simulink model "sim2_CompleteModel"  (R2014a)
settings: Solver=ode4  StartTime=0  StopTime=25  FixedStep=0.001  RelTol=1e-3
libraries: simulink x1
settings Model: Creator=Bruno  LastModifiedBy=Bruno
settings SolverCC: MaxConsecutiveZCs=100  ZeroCrossAlgorithm=Adaptive

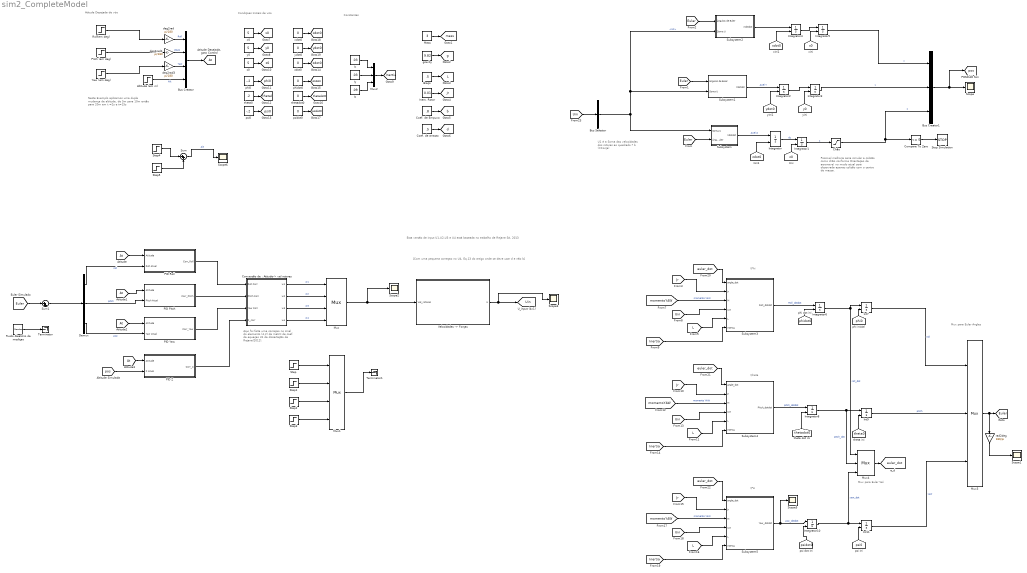
== system sim2_CompleteModel ==
  note: Aqui foi feita uma correçao no sinal do elemento (4,2) da matriz de coef. da equaçao 31 da dissertação de Rejane(2012).
  note: Neste Exemplo aplicamos uma dupla mudança de altitude, de 5m para 10m então para 20m em t =2s e t=15s
  note: Atitude Desejada de vôo
  note: Possível melhoria seria simular a colisão como chão conforme Orientaçao da aeronave! no modo atual será observada apenas colisão com o centro de massa.
  note: U1 é a Soma das velocidades dos rotores ao quadrado * b (=Força)
  note: \theta
  note: Mux para Euler Angles
  note: [Com uma pequena correçao no U4, Eq.13 do artigo onde se deve usar d e não b]
  note: Esta versão de input U1,U2,U3 e U4 está baseada no trabalho de Rejane Sá, 2013
  note: Constantes
  note: \Phi
  note: \Psi
  note: Mux para Euler Vel.
  note: Condiçoes Iniciais de vôo
  Altitude (em m) : Step  Time=0  Before=5  After=5  SampleTime=0
  Braço : Constant  Value=.5
  Bus Creator : BusCreator
  Bus Creator1 : BusCreator  Inputs=3
  Bus Selector : BusSelector  OutputSignals=U1
  Chão : Saturate  UpperLimit=inf  LowerLimit=-0.01
  Coef. de Empuxo : Constant  Value=.8
  Coef. de arrasto : Constant  Value=.5
  Compare To Zero : simulink/Logic and Bit Operations/Compare To Zero  relop=<=  OutDataTypeStr=boolean
  "Conversão de : Atitude-> vel rotores" : Subsystem
  Demux : Demux  Outputs=3
  Inerc. Rotor : Constant  Value=0.01
  Int11 : Integrator  InitialConditionSource=external
  Int7 : Integrator  InitialConditionSource=external
  Int9 : Integrator  InitialConditionSource=external
  Integrator : Integrator  InitialConditionSource=external  UpperSaturationLimit=1  LowerSaturationLimit=-1  IgnoreLimit=on
  Integrator1 : Integrator  InitialConditionSource=external  InitialCondition=20
  Integrator10 : Integrator  InitialConditionSource=external  UpperSaturationLimit=1  LowerSaturationLimit=-1  IgnoreLimit=on
  Integrator{2..6,8} (6 alike) : Integrator  InitialConditionSource=external
  Ix : Constant  Value=.03
  Iy : Constant  Value=.03
  Iz : Constant  Value=.09
  Mass : Constant  Value=3
  Mux : Mux
      settings: DisplayOption=signals
  Mux1 : Mux
      settings: DisplayOption=signals
  Mux2 : Mux  Inputs=3
  Mux3 : Mux  Inputs=3
      settings: DisplayOption=signals
  Mux4 : Mux  Inputs=3
      settings: DisplayOption=signals
  PID Pitch : Subsystem
  PID Roll : Subsystem
  PID Yaw : Subsystem
  PID Z : Subsystem
  Pitch (em deg) : Step  Time=0  After=0  SampleTime=0
  Roll(em deg) : Step  Time=0  After=0  SampleTime=0
  Ruído Aleatório da mediçao : UniformRandomNumber  Minimum=-.005  Maximum=.005  SampleTime=0
  Scope{,1..3,5..6} (6 alike) : Scope
      Scope settings: ShowLegends=on  YMin=3.95  SaveName=XYZ_Strategy1_C
      Scope1 settings: SaveName=Euler_Strategy1_C  Decimation=100
      Scope2 settings: ShowLegends=on  YMin=-1.1e+07  YMax=1.1e+07  SaveName=ScopeData3
      Scope3 settings: ShowLegends=on  YMin=0  YMax=1.3e+07  SaveName=ScopeData6
      Scope5 settings: ShowLegends=on  SaveName=ScopeData11
      Scope6 settings: ShowLegends=on  SaveName=ScopeData12
  Step{,1..3} (4 alike) : Step  Time=0  After=15  SampleTime=0
  Step4 : Step  Time=0  Before=5  After=5  SampleTime=0
  Step5 : Step  Time=5  SampleTime=0
  Stop Simulation : Stop
  Subsystem : Subsystem
  Subsystem1 : Subsystem
  Subsystem2 : Subsystem
  Subsystem3 : Subsystem
  Subsystem4 : Subsystem
  Subsystem5 : Subsystem
  Sum : Sum  Inputs=|++
  Sum1 : Sum  Inputs=|++
  Terminator : Terminator
  Terminator1 : Terminator
  "Velocidades -> Forças" : Subsystem
  Yaw (em deg) : Step  Time=0  After=0  SampleTime=0
  deg2rad : Gain  Gain=pi/180
  deg2rad2 : Gain  Gain=pi/180
  deg2rad3 : Gain  Gain=pi/180
  gravity : Constant  Value=9.82
  phi0 : Constant  Value=-.2
  phidot0 : Constant  Value=0
  psi0 : Constant  Value=-.2
  psidot0 : Constant  Value=0
  rad2deg : Gain  Gain=180/pi
  theta0 : Constant  Value=.2
  thetadot0 : Constant  Value=0
  x0 : Constant  Value=5
  xdot0 : Constant  Value=0
  y0 : Constant  Value=5
  ydot0 : Constant  Value=0
  z0 : Constant  Value=5
  zdot0 : Constant  Value=0
  tag scope: At=global, Euler=global, Inertia=global, Jr=global, L=global, Uin=global, b=global, d=global, euler_dot=global, g=global, mass=global, phi0=global, phidot0=global, pos=global, psi0=global, psidot0=global, theta0=global, thetadot0=global, x0=global, xdot0=global, y0=global, ydot0=global, z0=global, zdot0=global
  wires:
  Integrator/1 -> Integrator1/1  "dz"
  Integrator1/1 -> Chão/1  "z"
  Subsystem/1(zdotdot) -> Integrator/1  "Acel Z"
  Bus Selector/1 -> Subsystem/1(Soma U), Subsystem2/2(Soma U), Subsystem1/2(Soma U)  "<U1>"
  Subsystem1/1(Ydotdot) -> Integrator2/1  "Acel Y"
  Integrator2/1 -> Integrator3/1
  Subsystem2/1(Xdotdot) -> Integrator4/1
  Integrator4/1 -> Integrator5/1
  [Euler] -> Subsystem/2(Ângulos de Euler)
  [Euler] -> Subsystem1/1(ângulos de Euler)
  [Euler] -> Subsystem2/1(ângulos de Euler)
  Mass/1 -> [mass]
  gravity/1 -> [g]
  Braço/1 -> [L]
  [euler_dot] -> Subsystem3/1(angle_dot)
  [Jr] -> Subsystem3/2(Jr)
  [momentoYAW] -> Subsystem3/3(M)  "momento YAW"
  [Uin] -> Subsystem3/4(Uin)
  [L] -> Subsystem3/5(L)
  [Inertia] -> Subsystem3/6(Inertia)
  Subsystem3/1(Roll_dotdot) -> Integrator6/1  "Roll_dotdot"
  Inerc. Rotor/1 -> [Jr]
  Coef. de Empuxo/1 -> [b]
  Coef. de arrasto/1 -> [d]
  Iy/1 -> Mux2/2
  Ix/1 -> Mux2/1
  Iz/1 -> Mux2/3
  Mux2/1 -> [Inertia]
  Integrator6/1 -> Int7/1, Mux4/1  "roll_dot"
  Int7/1 -> Mux3/1  "roll"
  Mux3/1 -> [Euler], rad2deg/1
  [euler_dot] -> Subsystem4/1(angle_dot)
  [Jr] -> Subsystem4/2(Jr)
  [momentoYAW] -> Subsystem4/3(M)  "momento YAW"
  [Uin] -> Subsystem4/4(Uin)
  [L] -> Subsystem4/5(L)
  [Inertia] -> Subsystem4/6(Inertia)
  Subsystem4/1(Pitch_dotdot) -> Integrator8/1  "pitch_dotdot"
  Integrator8/1 -> Mux4/2, Int9/1  "pitch_dot"
  Int9/1 -> Mux3/2  "pitch"
  [euler_dot] -> Subsystem5/1(angle_dot)
  [Jr] -> Subsystem5/2(Jr)
  [momentoYAW] -> Subsystem5/3(M)  "momento YAW"
  [Uin] -> Subsystem5/4(Uin)
  [L] -> Subsystem5/5(L)
  [Inertia] -> Subsystem5/6(Inertia)
  Subsystem5/1(Yaw_dotdot) -> Scope5/1, Integrator10/1  "yaw_dotdot"
  Integrator10/1 -> Mux4/3, Int11/1  "yaw_dot"
  Int11/1 -> Mux3/3  "yaw"
  Mux4/1 -> [euler_dot]
  [Uin] -> Bus Selector/1
  Integrator3/1 -> Bus Creator1/2  "y"
  "Velocidades -> Forças"/1(U) -> Scope3/1, [Uin]
  [phi0] -> Int7/2
  [psi0] -> Int11/2
  [theta0] -> Int9/2
  x0/1 -> [x0]
  theta0/1 -> [theta0]
  psi0/1 -> [psi0]
  phi0/1 -> [phi0]
  z0/1 -> [z0]
  y0/1 -> [y0]
  xdot0/1 -> [xdot0]
  thetadot0/1 -> [thetadot0]
  psidot0/1 -> [psidot0]
  phidot0/1 -> [phidot0]
  zdot0/1 -> [zdot0]
  ydot0/1 -> [ydot0]
  [z0] -> Integrator1/2
  [phidot0] -> Integrator6/2
  [thetadot0] -> Integrator8/2
  [psidot0] -> Integrator10/2
  [zdot0] -> Integrator/2
  "Conversão de : Atitude-> vel rotores"/1(w1) -> Mux/1  "w1"
  "Conversão de : Atitude-> vel rotores"/3(w3) -> Mux/3  "w3"
  "Conversão de : Atitude-> vel rotores"/2(w2) -> Mux/2  "w2"
  "Conversão de : Atitude-> vel rotores"/4(w4) -> Mux/4  "w4"
  Chão/1 -> Bus Creator1/3, Compare To Zero/1  "z"
  Compare To Zero/1 -> Stop Simulation/1
  Roll(em deg)/1 -> deg2rad/1
  Pitch (em deg)/1 -> deg2rad2/1
  Yaw (em deg)/1 -> deg2rad3/1
  Bus Creator/1 -> [At]
  deg2rad/1 -> Bus Creator/1  "Roll"
  deg2rad2/1 -> Bus Creator/2  "Pitch"
  deg2rad3/1 -> Bus Creator/3  "Yaw"
  [At] -> PID Roll/1(Atitude)
  Demux/1 -> PID Roll/2(Roll Atual)  "roll"
  [At] -> PID Pitch/1(Atitude)
  Demux/2 -> PID Pitch/2(Pitch Atual)  "pitch"
  Demux/3 -> PID Yaw/2(Yaw Atual)  "yaw"
  [At] -> PID Yaw/1(Atitude)
  [At] -> PID Z/1(Atitude)
  Bus Creator1/1 -> [pos], Scope/1
  [pos] -> PID Z/2(Z Atual)
  PID Roll/1(Corr_Roll) -> "Conversão de : Atitude-> vel rotores"/1(Roll Corr)
  PID Pitch/1(Corr_Pitch) -> "Conversão de : Atitude-> vel rotores"/2(Pitch Corr)
  PID Yaw/1(Corr_Yaw) -> "Conversão de : Atitude-> vel rotores"/3(Yaw Corr)
  PID Z/1(Corr_Z) -> "Conversão de : Atitude-> vel rotores"/4(Z_corr)
  Step4/1 -> Sum/1
  Step5/1 -> Sum/2
  Sum/1 -> Scope6/1  "Alt"
  Altitude (em m)/1 -> Bus Creator/4  "Alt"
  Integrator5/1 -> Bus Creator1/1  "x"
  [x0] -> Integrator5/2
  [xdot0] -> Integrator4/2
  [ydot0] -> Integrator2/2
  [y0] -> Integrator3/2
  Mux/1 -> "Velocidades -> Forças"/1(Vel_rotores), Scope2/1
  rad2deg/1 -> Scope1/1
  [Euler] -> Sum1/1
  Ruído Aleatório da mediçao/1 -> Terminator/1
  Sum1/1 -> Demux/1
  Step2/1 -> Mux1/3
  Step1/1 -> Mux1/2
  Step/1 -> Mux1/1
  Step3/1 -> Mux1/4
  Mux1/1 -> Terminator1/1

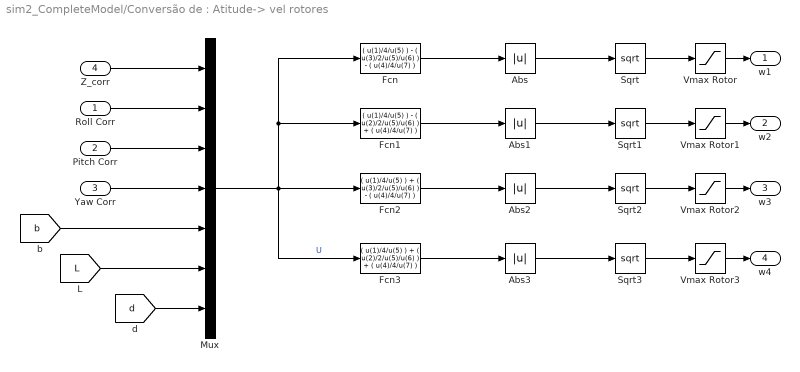
== system sim2_CompleteModel/Conversão de : Atitude-> vel rotores ==
  Roll Corr : Inport
  Pitch Corr : Inport  Port=2
  Yaw Corr : Inport  Port=3
  Z_corr : Inport  Port=4
  Abs{,1..3} (4 alike) : Abs
  Fcn : Fcn  Expr="( u(1)/4/u(5) ) - ( u(3)/2/u(5)/u(6) )  - ( u(4)/4/u(7) )"
  Fcn1 : Fcn  Expr="( u(1)/4/u(5) ) - ( u(2)/2/u(5)/u(6) )  + ( u(4)/4/u(7) )"
  Fcn2 : Fcn  Expr="( u(1)/4/u(5) ) + ( u(3)/2/u(5)/u(6) )  - ( u(4)/4/u(7) )"
  Fcn3 : Fcn  Expr="( u(1)/4/u(5) ) + ( u(2)/2/u(5)/u(6) )  + ( u(4)/4/u(7) )"
  Mux : Mux  Inputs=7
  Sqrt{,1..3} (4 alike) : Sqrt  SaturateOnIntegerOverflow=on
  Vmax Rotor{,1..3} (4 alike) : Saturate  UpperLimit=10  LowerLimit=-10
  w1 : Outport
  w2 : Outport  Port=2
  w3 : Outport  Port=3
  w4 : Outport  Port=4
  wires:
  Mux/1 -> Fcn1/1, Fcn/1, Fcn3/1, Fcn2/1  "U"
  [L] -> Mux/6
  [b] -> Mux/5
  [d] -> Mux/7
  Fcn/1 -> Abs/1
  Sqrt/1 -> Vmax Rotor/1
  Fcn1/1 -> Abs1/1
  Fcn2/1 -> Abs2/1
  Fcn3/1 -> Abs3/1
  Sqrt1/1 -> Vmax Rotor1/1
  Sqrt2/1 -> Vmax Rotor2/1
  Sqrt3/1 -> Vmax Rotor3/1
  Abs/1 -> Sqrt/1
  Abs1/1 -> Sqrt1/1
  Abs2/1 -> Sqrt2/1
  Abs3/1 -> Sqrt3/1
  Vmax Rotor/1 -> w1/1
  Vmax Rotor1/1 -> w2/1
  Vmax Rotor2/1 -> w3/1
  Vmax Rotor3/1 -> w4/1
  Z_corr/1 -> Mux/1
  Roll Corr/1 -> Mux/2
  Pitch Corr/1 -> Mux/3
  Yaw Corr/1 -> Mux/4

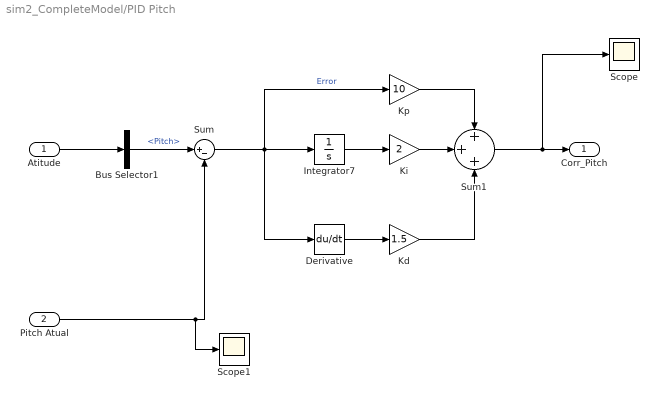
== system sim2_CompleteModel/PID Pitch ==
  Atitude : Inport
  Pitch Atual : Inport  Port=2
  Bus Selector1 : BusSelector  OutputSignals=Pitch
  Derivative : Derivative
  Integrator7 : Integrator  UpperSaturationLimit=1  LowerSaturationLimit=-1
  Kd : Gain  Gain=1.5
  Ki : Gain  Gain=2
  Kp : Gain  Gain=10
  Scope : Scope
      settings: SaveName=ScopeData4
  Scope1 : Scope
      settings: ShowLegends=on  SaveName=ScopeData9
  Sum : Sum  Inputs=|+-
  Sum1 : Sum  Inputs=+++
  Corr_Pitch : Outport
  wires:
  Bus Selector1/1 -> Sum/1  "<Pitch>"
  Ki/1 -> Sum1/2
  Sum/1 -> Derivative/1, Integrator7/1, Kp/1  "Error"
  Derivative/1 -> Kd/1
  Pitch Atual/1 -> Scope1/1, Sum/2
  Kp/1 -> Sum1/1
  Kd/1 -> Sum1/3
  Sum1/1 -> Scope/1, Corr_Pitch/1
  Atitude/1 -> Bus Selector1/1
  Integrator7/1 -> Ki/1

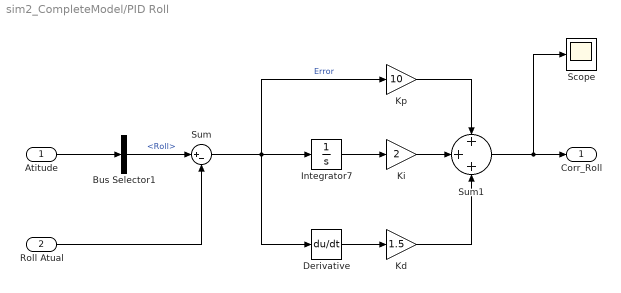
== system sim2_CompleteModel/PID Roll ==
  Atitude : Inport
  Roll Atual : Inport  Port=2
  Bus Selector1 : BusSelector  OutputSignals=Roll
  Derivative : Derivative
  Integrator7 : Integrator  UpperSaturationLimit=1  LowerSaturationLimit=-1
  Kd : Gain  Gain=1.5
  Ki : Gain  Gain=2
  Kp : Gain  Gain=10
  Scope : Scope
      settings: ShowLegends=on  SaveName=ScopeData8
  Sum : Sum  Inputs=|+-
  Sum1 : Sum  Inputs=+++
  Corr_Roll : Outport
  wires:
  Bus Selector1/1 -> Sum/1  "<Roll>"
  Ki/1 -> Sum1/2
  Sum/1 -> Derivative/1, Integrator7/1, Kp/1  "Error"
  Derivative/1 -> Kd/1
  Roll Atual/1 -> Sum/2
  Kp/1 -> Sum1/1
  Kd/1 -> Sum1/3
  Sum1/1 -> Scope/1, Corr_Roll/1
  Atitude/1 -> Bus Selector1/1
  Integrator7/1 -> Ki/1

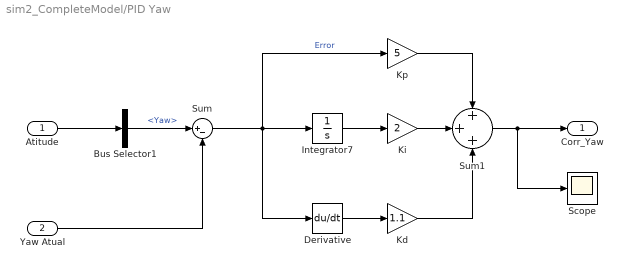
== system sim2_CompleteModel/PID Yaw ==
  Atitude : Inport
  Yaw Atual : Inport  Port=2
  Bus Selector1 : BusSelector  OutputSignals=Yaw
  Derivative : Derivative
  Integrator7 : Integrator  UpperSaturationLimit=1  LowerSaturationLimit=-1
  Kd : Gain  Gain=1.1
  Ki : Gain  Gain=2
  Kp : Gain  Gain=5
  Scope : Scope
      settings: SaveName=ScopeData13
  Sum : Sum  Inputs=|+-
  Sum1 : Sum  Inputs=+++
  Corr_Yaw : Outport
  wires:
  Integrator7/1 -> Ki/1
  Atitude/1 -> Bus Selector1/1
  Sum1/1 -> Scope/1, Corr_Yaw/1
  Kd/1 -> Sum1/3
  Kp/1 -> Sum1/1
  Yaw Atual/1 -> Sum/2
  Derivative/1 -> Kd/1
  Sum/1 -> Kp/1, Integrator7/1, Derivative/1  "Error"
  Ki/1 -> Sum1/2
  Bus Selector1/1 -> Sum/1  "<Yaw>"

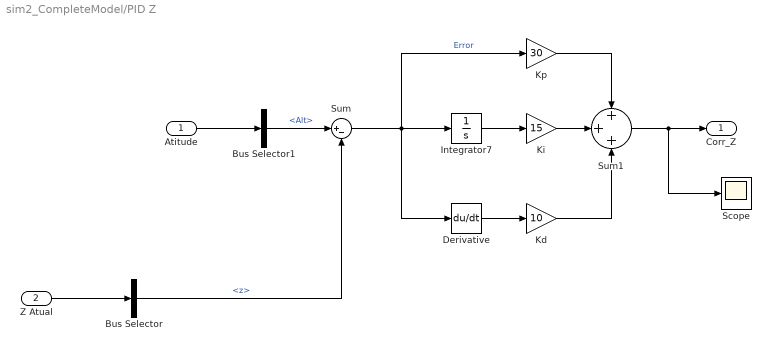
== system sim2_CompleteModel/PID Z ==
  Atitude : Inport
  Z Atual : Inport  Port=2
  Bus Selector : BusSelector  OutputSignals=z
  Bus Selector1 : BusSelector  OutputSignals=Alt
  Derivative : Derivative
  Integrator7 : Integrator  UpperSaturationLimit=1  LowerSaturationLimit=-1
  Kd : Gain  Gain=10
  Ki : Gain  Gain=15
  Kp : Gain  Gain=30
  Scope : Scope
      settings: YMin=27.1  YMax=28  SaveName=ScopeData5
  Sum : Sum  Inputs=|+-
  Sum1 : Sum  Inputs=+++
  Corr_Z : Outport
  wires:
  Bus Selector1/1 -> Sum/1  "<Alt>"
  Ki/1 -> Sum1/2
  Sum/1 -> Derivative/1, Integrator7/1, Kp/1  "Error"
  Derivative/1 -> Kd/1
  Kp/1 -> Sum1/1
  Kd/1 -> Sum1/3
  Sum1/1 -> Scope/1, Corr_Z/1
  Atitude/1 -> Bus Selector1/1
  Integrator7/1 -> Ki/1
  Z Atual/1 -> Bus Selector/1
  Bus Selector/1 -> Sum/2  "<z>"

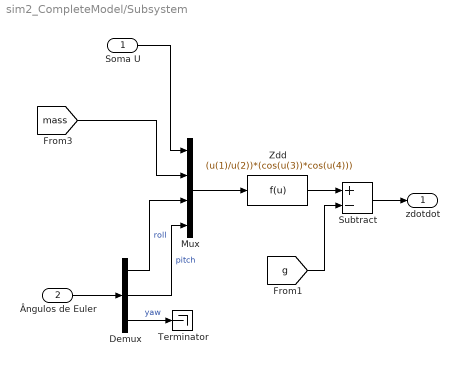
== system sim2_CompleteModel/Subsystem ==
  Soma U : Inport
  Ângulos de Euler : Inport  Port=2
  Demux : Demux  Outputs=3
  Mux : Mux
  Subtract : Sum  Inputs=+-
  Terminator : Terminator
  Zdd : Fcn  Expr=(u(1)/u(2))*(cos(u(3))*cos(u(4)))
  zdotdot : Outport
  wires:
  Soma U/1 -> Mux/1
  Demux/1 -> Mux/3  "roll"
  Mux/1 -> Zdd/1
  Demux/3 -> Terminator/1  "yaw"
  [mass] -> Mux/2
  Demux/2 -> Mux/4  "pitch"
  Ângulos de Euler/1 -> Demux/1
  Zdd/1 -> Subtract/1
  Subtract/1 -> zdotdot/1
  [g] -> Subtract/2

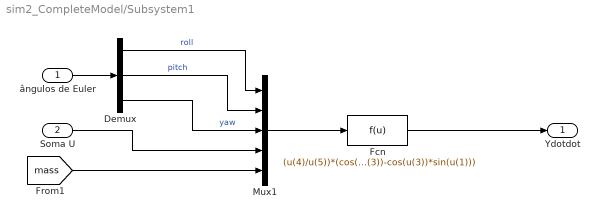
== system sim2_CompleteModel/Subsystem1 ==
  ângulos de Euler : Inport
  Soma U : Inport  Port=2
  Demux : Demux  Outputs=3
  Fcn : Fcn  Expr=(u(4)/u(5))*(cos(u(1))*sin(u(2))*sin(u(3))-cos(u(3))*sin(u(1)))
  Mux1 : Mux  Inputs=5
  Ydotdot : Outport
  wires:
  Demux/3 -> Mux1/3  "yaw"
  Demux/2 -> Mux1/2  "pitch"
  Mux1/1 -> Fcn/1
  Fcn/1 -> Ydotdot/1
  ângulos de Euler/1 -> Demux/1
  Demux/1 -> Mux1/1  "roll"
  [mass] -> Mux1/5
  Soma U/1 -> Mux1/4

== system sim2_CompleteModel/Subsystem2 ==
  ângulos de Euler : Inport
  Soma U : Inport  Port=2
  Demux : Demux  Outputs=3
  Fcn : Fcn  Expr=(u(4)/u(5))*(sin(u(1))*sin(u(3))+cos(u(1))*cos(u(3))*sin(u(2)))
  Mux1 : Mux  Inputs=5
  Xdotdot : Outport
  wires:
  Soma U/1 -> Mux1/4
  [mass] -> Mux1/5
  Demux/1 -> Mux1/1  "roll"
  ângulos de Euler/1 -> Demux/1
  Fcn/1 -> Xdotdot/1
  Mux1/1 -> Fcn/1
  Demux/2 -> Mux1/2  "pitch"
  Demux/3 -> Mux1/3  "yaw"

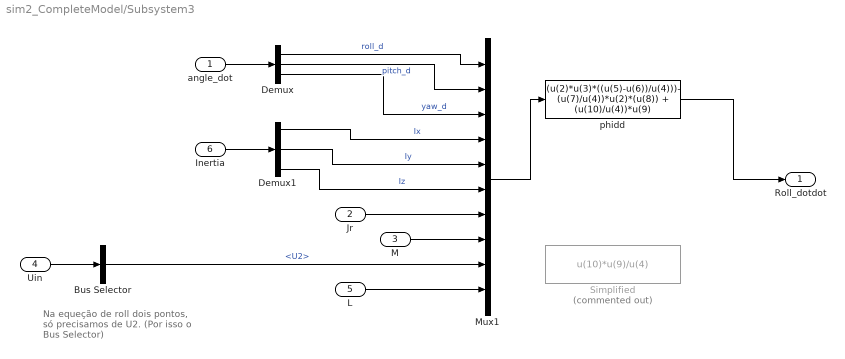
== system sim2_CompleteModel/Subsystem3 ==
  note: Na equeção de roll dois pontos, só precisamos de U2.
      |  (Por isso o Bus Selector)
  angle_dot : Inport
  Jr : Inport  Port=2
  M : Inport  Port=3
  Uin : Inport  Port=4
  L : Inport  Port=5
  Inertia : Inport  Port=6
  Bus Selector : BusSelector  OutputSignals=U2
  Demux : Demux  Outputs=3
  Demux1 : Demux  Outputs=3
  Mux1 : Mux  Inputs=10
  Simplified : Fcn  Commented=on  Expr=u(10)*u(9)/u(4)
  phidd : Fcn  Expr=(u(2)*u(3)*((u(5)-u(6))/u(4)))- (u(7)/u(4))*u(2)*(u(8)) + (u(10)/u(4))*u(9)
  Roll_dotdot : Outport
  wires:
  Demux1/1 -> Mux1/4  "Ix"
  Demux1/2 -> Mux1/5  "Iy"
  Mux1/1 -> phidd/1
  angle_dot/1 -> Demux/1
  M/1 -> Mux1/8
  Demux/2 -> Mux1/2  "pitch_d"
  Demux/1 -> Mux1/1  "roll_d"
  Demux/3 -> Mux1/3  "yaw_d"
  Inertia/1 -> Demux1/1
  Jr/1 -> Mux1/7
  L/1 -> Mux1/10
  Demux1/3 -> Mux1/6  "Iz"
  Uin/1 -> Bus Selector/1
  Bus Selector/1 -> Mux1/9  "<U2>"
  phidd/1 -> Roll_dotdot/1

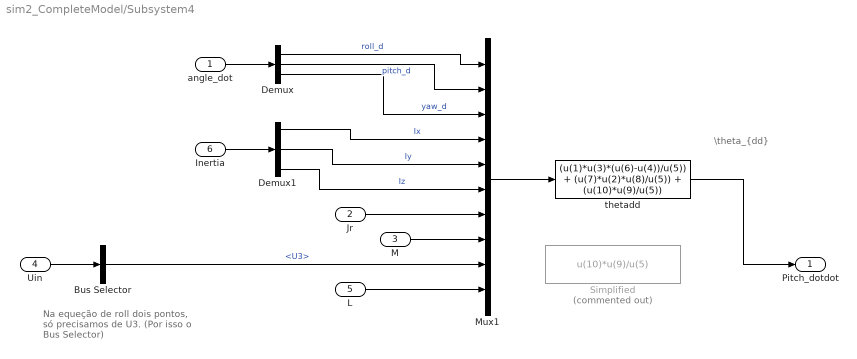
== system sim2_CompleteModel/Subsystem4 ==
  note: \theta_{dd}
  note: Na equeção de roll dois pontos, só precisamos de U3.
      |  (Por isso o Bus Selector)
  angle_dot : Inport
  Jr : Inport  Port=2
  M : Inport  Port=3
  Uin : Inport  Port=4
  L : Inport  Port=5
  Inertia : Inport  Port=6
  Bus Selector : BusSelector  OutputSignals=U3
  Demux : Demux  Outputs=3
  Demux1 : Demux  Outputs=3
  Mux1 : Mux  Inputs=10
  Simplified : Fcn  Commented=on  Expr=u(10)*u(9)/u(5)
  thetadd : Fcn  Expr=(u(1)*u(3)*(u(6)-u(4))/u(5)) + (u(7)*u(2)*u(8)/u(5)) + (u(10)*u(9)/u(5))
  Pitch_dotdot : Outport
  wires:
  Bus Selector/1 -> Mux1/9  "<U3>"
  Uin/1 -> Bus Selector/1
  Demux1/3 -> Mux1/6  "Iz"
  L/1 -> Mux1/10
  Jr/1 -> Mux1/7
  Inertia/1 -> Demux1/1
  Demux/3 -> Mux1/3  "yaw_d"
  Demux/1 -> Mux1/1  "roll_d"
  Demux/2 -> Mux1/2  "pitch_d"
  M/1 -> Mux1/8
  angle_dot/1 -> Demux/1
  Mux1/1 -> thetadd/1
  Demux1/2 -> Mux1/5  "Iy"
  Demux1/1 -> Mux1/4  "Ix"
  thetadd/1 -> Pitch_dotdot/1

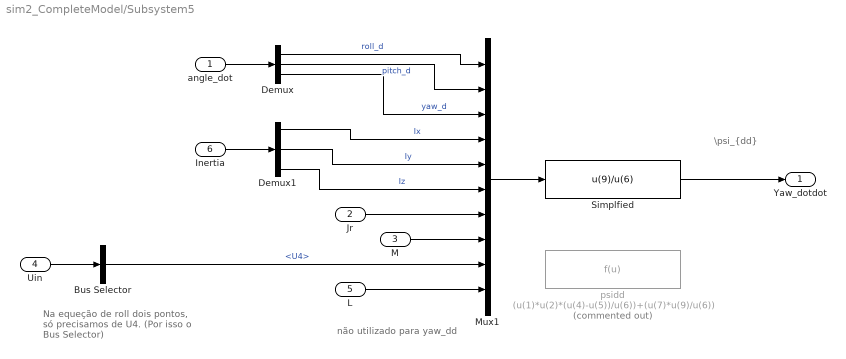
== system sim2_CompleteModel/Subsystem5 ==
  note: não utilizado para yaw_dd
  note: \psi_{dd}
  note: Na equeção de roll dois pontos, só precisamos de U4.
      |  (Por isso o Bus Selector)
  angle_dot : Inport
  Jr : Inport  Port=2
  M : Inport  Port=3
  Uin : Inport  Port=4
  L : Inport  Port=5
  Inertia : Inport  Port=6
  Bus Selector : BusSelector  OutputSignals=U4
  Demux : Demux  Outputs=3
  Demux1 : Demux  Outputs=3
  Mux1 : Mux  Inputs=10
  Simplfied : Fcn  Expr=u(9)/u(6)
  psidd : Fcn  Commented=on  Expr=(u(1)*u(2)*(u(4)-u(5))/u(6))+(u(7)*u(9)/u(6))
  Yaw_dotdot : Outport
  wires:
  Bus Selector/1 -> Mux1/9  "<U4>"
  Uin/1 -> Bus Selector/1
  Demux1/3 -> Mux1/6  "Iz"
  L/1 -> Mux1/10
  Jr/1 -> Mux1/7
  Inertia/1 -> Demux1/1
  Demux/3 -> Mux1/3  "yaw_d"
  Demux/1 -> Mux1/1  "roll_d"
  Demux/2 -> Mux1/2  "pitch_d"
  M/1 -> Mux1/8
  angle_dot/1 -> Demux/1
  Mux1/1 -> Simplfied/1
  Demux1/2 -> Mux1/5  "Iy"
  Demux1/1 -> Mux1/4  "Ix"
  Simplfied/1 -> Yaw_dotdot/1

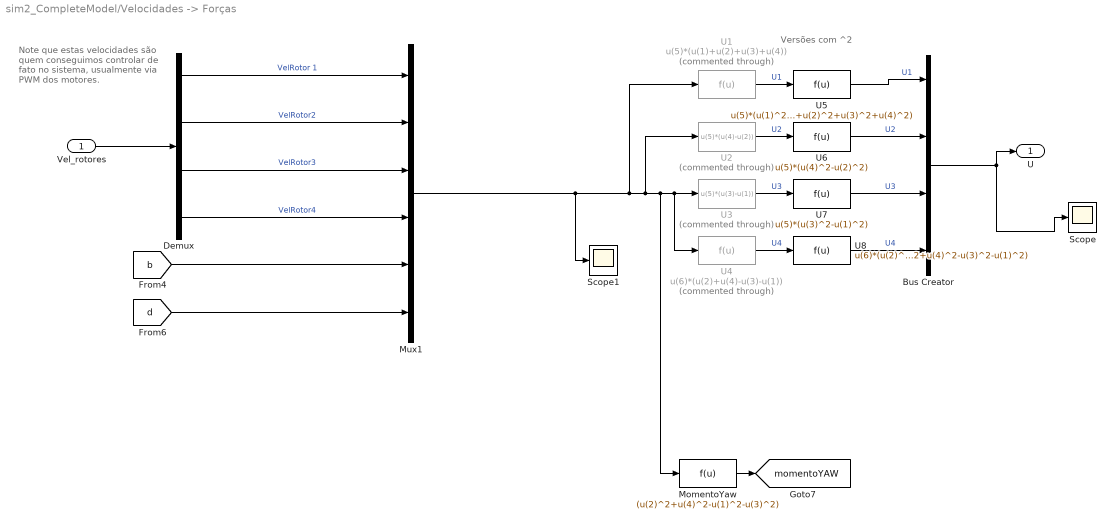
== system sim2_CompleteModel/Velocidades -> Forças ==
  note: Versões com ^2
  note: Note que estas velocidades são quem conseguimos controlar de fato no sistema, usualmente via PWM dos motores.
  Vel_rotores : Inport
  Bus Creator : BusCreator
  Demux : Demux
  MomentoYaw : Fcn  Expr=(u(2)^2+u(4)^2-u(1)^2-u(3)^2)
  Mux1 : Mux  Inputs=6
  Scope : Scope
      settings: ShowLegends=on  SaveName=ScopeData2
  Scope1 : Scope
      settings: ShowLegends=on  SaveName=ScopeData7
  U1 : Fcn  Commented=through  Expr=u(5)*(u(1)+u(2)+u(3)+u(4))
  U2 : Fcn  Commented=through  Expr=u(5)*(u(4)-u(2))
  U3 : Fcn  Commented=through  Expr=u(5)*(u(3)-u(1))
  U4 : Fcn  Commented=through  Expr=u(6)*(u(2)+u(4)-u(3)-u(1))
  U5 : Fcn  Expr=u(5)*(u(1)^2+u(2)^2+u(3)^2+u(4)^2)
  U6 : Fcn  Expr=u(5)*(u(4)^2-u(2)^2)
  U7 : Fcn  Expr=u(5)*(u(3)^2-u(1)^2)
  U8 : Fcn  Expr=u(6)*(u(2)^2+u(4)^2-u(3)^2-u(1)^2)
  U : Outport
  tag scope: momentoYAW=global
  wires:
  U3/1 -> U7/1  "U3"
  Demux/3 -> Mux1/3  "VelRotor3"
  Demux/4 -> Mux1/4  "VelRotor4"
  Demux/2 -> Mux1/2  "VelRotor2"
  Demux/1 -> Mux1/1  "VelRotor 1"
  Vel_rotores/1 -> Demux/1
  [b] -> Mux1/5
  [d] -> Mux1/6
  U4/1 -> U8/1  "U4"
  U1/1 -> U5/1  "U1"
  U2/1 -> U6/1  "U2"
  MomentoYaw/1 -> [momentoYAW]
  Bus Creator/1 -> Scope/1, U/1
  Mux1/1 -> Scope1/1, U4/1, U3/1, MomentoYaw/1, U2/1, U1/1
  U5/1 -> Bus Creator/1  "U1"
  U7/1 -> Bus Creator/3  "U3"
  U6/1 -> Bus Creator/2  "U2"
  U8/1 -> Bus Creator/4  "U4"
